simulink model "arm"  (R2019b)
settings: Solver=VariableStepAuto  StartTime=0.0  StopTime=10.0  RelTol=1e-3
values from neighbouring files (symbols this model uses):
  a = 1    [arm_model_runner.m]
  m = .5    (= 0.5)    [arm_model_runner.m]
  M = 1.5    [arm_model_runner.m]
  mu = 1    [arm_model_runner.m]
settings Model: Creator=nathanielgoldfarb  LastModifiedBy=nathanielgoldfarb

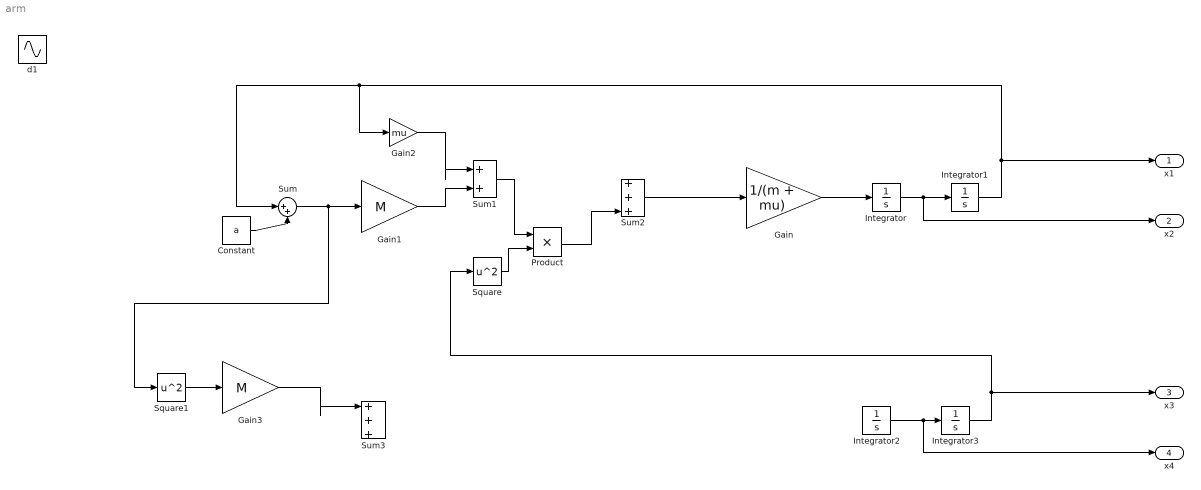
== system arm ==
  Constant : Constant  Value=a
  Gain : Gain  Gain=1/(m + mu)
  Gain1 : Gain  Gain=M
  Gain2 : Gain  Gain=mu
  Gain3 : Gain  Gain=M
  Integrator{,1..3} (4 alike) : Integrator
  Product : Product
  Square : Math  Operator=square  SignedPower=off  SaturateOnIntegerOverflow=on
  Square1 : Math  Operator=square  SignedPower=off  SaturateOnIntegerOverflow=on
  Sum : Sum  Inputs=|++
  Sum1 : Sum  Inputs=|++
  Sum2 : Sum  Inputs=|+++
  Sum3 : Sum  Inputs=|+++
  d1 : Sin  Amplitude=0.3  Frequency=4  Phase=0.5*pi  SampleTime=0
  x1 : Outport
  x2 : Outport  Port=2
  x3 : Outport  Port=3
  x4 : Outport  Port=4
  wires:
  Constant/1 -> Sum/2
  Sum/1 -> Square1/1, Gain1/1
  Integrator1/1 -> x1/1, Gain2/1, Sum/1
  Gain1/1 -> Sum1/2
  Gain2/1 -> Sum1/1
  Sum1/1 -> Product/1
  Square/1 -> Product/2
  Gain/1 -> Integrator/1
  Product/1 -> Sum2/3
  Sum2/1 -> Gain/1
  Integrator/1 -> x2/1, Integrator1/1
  Integrator2/1 -> x4/1, Integrator3/1
  Integrator3/1 -> x3/1, Square/1
  ? -> Integrator2/1
  Square1/1 -> Gain3/1
  Gain3/1 -> Sum3/1
